simulink model "gm_base_band_shaping_model_fil"  (R2020b)
settings: Solver=FixedStepDiscrete  StartTime=0.0  StopTime=400  RelTol=1e-3
libraries: simulink x2, dspmlti4 x2, whdlio x1, commdigbbndpm3 x1, commrandsrc3 x1, fillib x1
settings Model: Creator=wardo  LastModifiedBy=wardo
settings DataIOCC: LimitDataPoints=on  SaveOutput=off  SaveTime=off
settings OptimizationCC: BlockReduction=off  ConditionallyExecuteInputs=off  DefaultParameterBehavior=Inlined  LifeSpan=inf
settings DebuggingCC: AlgebraicLoopMsg=error  InheritedTsInSrcMsg=none  SingleTaskRateTransMsg=error  AllowSymbolicDim=off  StrictBusMsg=ErrorOnBusTreatedAsVector  SFUnexpectedBacktrackingDiag=warning  SFNoUnconditionalDefaultTransitionDiag=warning  SFExecutionAtInitializationDiag=none  ArithmeticOperatorsInVariantConditions=warning
settings HardwareCC: ProdBitPerPointer=32  ProdBitPerSizeT=32  ProdBitPerPtrDiffT=32  ProdLargestAtomicFloat=None  ProdIntDivRoundTo=Undefined  ProdEndianess=Unspecified  ProdWordSize=32  ProdHWDeviceType=ASIC/FPGA->ASIC/FPGA  ProdEqTarget=off
settings SFSimCC: SimUseLocalCustomCode=off  CustomCodeUndefinedFunction=UseInterfaceOnly
settings RTWCC: RTWUseLocalCustomCode=off
settings CodeAppCC: StateflowObjectComments=on
settings GRTTargetCC: TargetLangStandard=C89/C90 (ANSI)
settings ConfigComp: CovScope=ReferencedModels  CovMetricSettings=dw  CovSaveCumulativeToWorkspaceVar=on  CovSaveSingleToWorkspaceVar=on  CovExternalEMLEnable=off  CovSFcnEnable=off

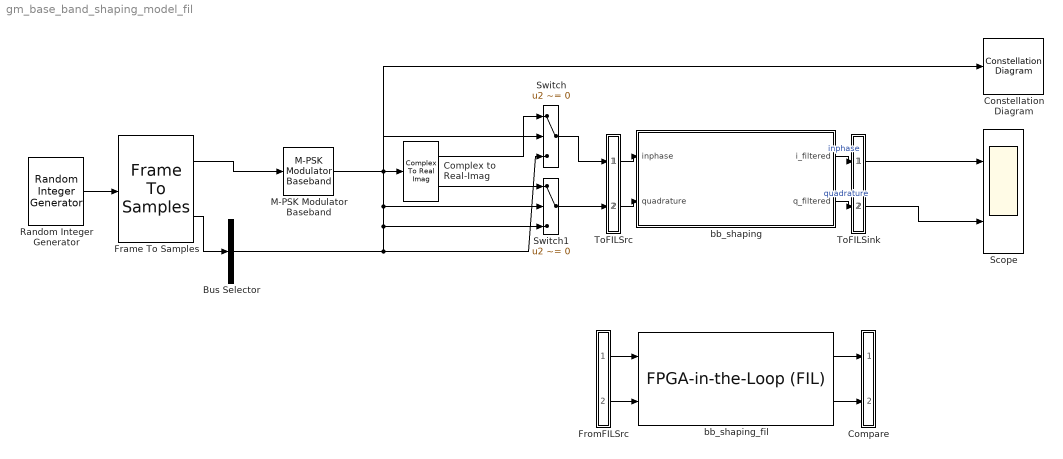
== system gm_base_band_shaping_model_fil ==
  Bus Selector : BusSelector  OutputSignals=valid
  Compare : Subsystem
      mask Display: disp('')
  Complex to Real-Imag : ComplexToRealImag
  Constellation Diagram : ConstellationDiagram
  Frame To Samples : whdlio/Frame To Samples  InterSampleIdleCycles=1  InterFrameIdleCycles=100  OutputSize=1  InterleaveSamples=off
      settings: SourceProductBaseCode=LH
  FromFILSrc : Subsystem
      mask Display: disp('')
  M-PSK Modulator Baseband : commdigbbndpm3/M-PSK Modulator Baseband  M=8  InType=Integer  Enc=Gray  Mapping=[0:7]  Ph=0  outDtype=Fixed-point  outWordLen=18  outUDDataType=sfix(16)  outFracLenMode=User-defined  outFracLen=14  outDataTypeStr=fixdt(1,18,14)  outLastDataTypeStr=fixdt(1,18,14)
      settings: SourceProductName=Communications Toolbox
  Random Integer Generator : commrandsrc3/Random Integer Generator  SetSize=8  SeedSource=Auto  Seed=0  SampleTime=10  SamplesPerFrame=10  OutputDataType=double  SimulateUsing=Interpreted execution
  Scope : Scope  NumInputPorts=2
  Switch : Switch  Criteria=u2 ~= 0  OutDataTypeStr=Inherit: Inherit via back propagation
  Switch1 : Switch  Criteria=u2 ~= 0  OutDataTypeStr=Inherit: Inherit via back propagation
  ToFILSink : Subsystem
      mask Display: disp('')
  ToFILSrc : Subsystem
      mask Display: disp('')
  bb_shaping : Subsystem
  bb_shaping_fil : fillib/FPGA-in-the-Loop (FIL)  ForceInterfaceUpdate=0.43904
      settings: SourceProductBaseCode=ES,HD
  wires:
  Frame To Samples/1 -> M-PSK Modulator Baseband/1
  M-PSK Modulator Baseband/1 -> Complex to Real-Imag/1, Constellation Diagram/1
  Random Integer Generator/1 -> Frame To Samples/1
  Frame To Samples/2 -> Bus Selector/1
  Bus Selector/1 -> Switch/2, Switch1/2, Switch1/3, Switch/3
  Complex to Real-Imag/1 -> Switch/1
  Complex to Real-Imag/2 -> Switch1/1
  ToFILSrc/1(out1) -> bb_shaping/1(inphase)
  ToFILSrc/2(out2) -> bb_shaping/2(quadrature)
  bb_shaping/1(i_filtered) -> ToFILSink/1(in1)  "inphase"
  bb_shaping/2(q_filtered) -> ToFILSink/2(in2)  "quadrature"
  Switch/1 -> ToFILSrc/1(in1)
  Switch1/1 -> ToFILSrc/2(in2)
  ToFILSink/1(out1) -> Scope/1
  ToFILSink/2(out2) -> Scope/2
  FromFILSrc/1(out1) -> bb_shaping_fil/1
  FromFILSrc/2(out2) -> bb_shaping_fil/2
  bb_shaping_fil/1 -> Compare/1(in1)
  bb_shaping_fil/2 -> Compare/2(in2)

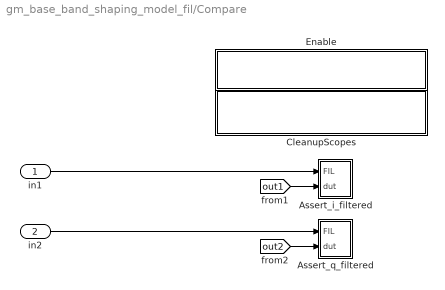
== system gm_base_band_shaping_model_fil/Compare ==
  in1 : Inport
  in2 : Inport  Port=2
  Assert_i_filtered : Subsystem
  Assert_q_filtered : Subsystem
  CleanupScopes : Subsystem
      settings: OpenFcn=|
      | blkName = gcb; %self block
      | idx = regexp(blkName, '/CleanupScopes$', 'once');
      | blkParent = blkName(1:idx-1);
      | blks=find_system(blkParent, 'LookUnderMasks', 'all','blocktype', 'Scope');
      | for itr = 1:length(blks)
      | 	 hScopeCfg = get_param(blks{itr},'ScopeConfiguration');
      | 	 hScopeCfg.Visible = ~ hScopeCfg.Visible;
      | end
      | drawnow;
      mask Display: fprintf(message('hdlcoder:cosim:vnl_dblclick').getString());
  Enable : Subsystem
      settings: OpenFcn=|
      | blkName = gcb;
      | idx = regexp(blkName, '/Enable$', 'once');
      | blkParent = blkName(1:idx-1);
      | blks=find_system(blkParent, 'LookUnderMasks', 'all','blocktype', 'Assertion');
      | e = get_param(blks{1}, 'Enabled');
      | if strcmp(e, 'on'), f= 'off';, else, f = 'on';, end
      | for ii=1:length(blks), set_param(blks{ii}, 'Enabled', f);, end
      | set_param(gcb, 'MaskDisplay',['fprintf(message(''hdlcoder:cosim:vnl_dblclick_assertions'',','''',upper(e),'''',').getString())']);
      mask Display: fprintf(message('hdlcoder:cosim:vnl_dblclick_assertions','OFF').getString());
  wires:
  in1/1 -> Assert_i_filtered/1(FIL)
  [out1] -> Assert_i_filtered/2(dut)
  in2/1 -> Assert_q_filtered/1(FIL)
  [out2] -> Assert_q_filtered/2(dut)

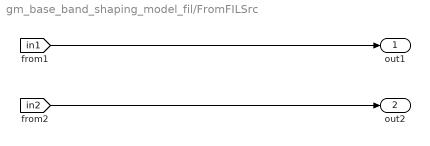
== system gm_base_band_shaping_model_fil/FromFILSrc ==
  out1 : Outport
  out2 : Outport  Port=2
  wires:
  [in1] -> out1/1
  [in2] -> out2/1

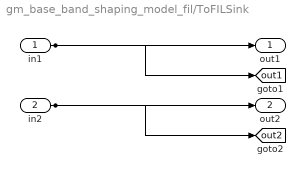
== system gm_base_band_shaping_model_fil/ToFILSink ==
  in1 : Inport
  in2 : Inport  Port=2
  out1 : Outport
  out2 : Outport  Port=2
  tag scope: out1=global, out2=global
  wires:
  in1/1 -> out1/1, [out1]
  in2/1 -> out2/1, [out2]

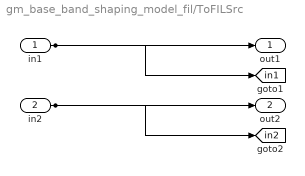
== system gm_base_band_shaping_model_fil/ToFILSrc ==
  in1 : Inport
  in2 : Inport  Port=2
  out1 : Outport
  out2 : Outport  Port=2
  tag scope: in1=global, in2=global
  wires:
  in1/1 -> out1/1, [in1]
  in2/1 -> out2/1, [in2]

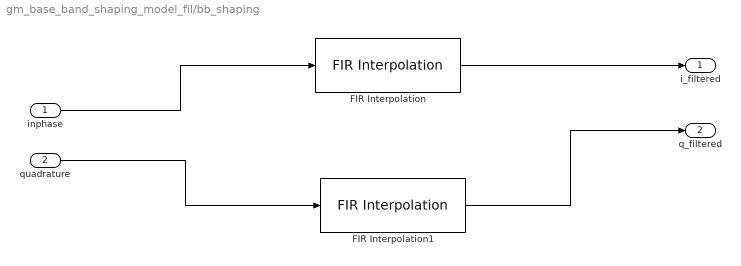
== system gm_base_band_shaping_model_fil/bb_shaping ==
  inphase : Inport  OutDataTypeStr=fixdt(1, 18, 14)  PortDimensions=1  SampleTime=0.833333333333333
  quadrature : Inport  Port=2  OutDataTypeStr=fixdt(1, 18, 14)  PortDimensions=1  SampleTime=0.833333333333333
  FIR Interpolation : dspmlti4/FIR Interpolation  FilterSource=Dialog parameters  PrivateCoeffs=0  h=[-0.00599670410156250,-0.00514221191406250,-0.00289916992187500,0.000442504882812500,0.00431823730468750,0.00794982910156250,0.0104980468750000,0.0112304687500000,0.00967407226562500,0.00578308105468750,0,-0.00680541992187500,-0.0134124755859375,-0.0184326171875000,-0.0205841064453125,-0.0189819335937500,-0.0133361816406250,-0.00410461425781250,0.00752258300781250,0.0196380615234375,0.0300140380859375,0.0363464355468750,0.0367584228515625,0.0301208496093750,0.0164794921875000,-0.00291442871093750,-0.0254821777343750,-0.0476837158203125,-0.0653228759765625,-0.0742187500000000,-0.0707244873046875,-0.0524291992187500,-0.0185852050781250,0.0296783447265625,0.0892028808593750,0.155227661132813,0.221755981445313,0.282333374023438,0.330810546875000,0.362121582031250,0.372940063476563,0.362121582031250,0.330810546875000,0.282333374023438,0.221755981445313,0.155227661132813,0.0892028808593750,0.0296783447265625,-0.0185852050781250,-0.0524291992187500,-0.0707244873046875,-0.0742187500000000,-0.0653228759765625,-0.0476837158203125,-0.0254821777343750,-0.00291442871093750,0.0164794921875000,0.0301208496093750,0.0367584228515625,0.0363464355468750,0.0300140380859375,0.0196380615234375,0.00752258300781250,-0.00410461425781250,-0.0133361816406250,-0.0189819335937500,-0.0205841064453125,-0.0184326171875000,-0.0134124755859375,-0.00680541992187500,0,0.00578308105468750,0.00967407226562500,0.0112304687500000,0.0104980468750000,0.00794982910156250,0.00431823730468750,0.000442504882812500,-0.00289916992187500,-0.00514221191406250,-0.00599670410156250]  L=8  FilterObject=FINTERP  framing=Allow multirate processing  outputBufInitCond=0  roundingMode=Floor  overflowMode=off  firstCoeffMode=Specify word length  firstCoeffWordLength=16  firstCoeffFracLength=15  firstCoeffDataTypeStr=fixdt(1,16)  firstCoeffMin=[]  firstCoeffMax=[]  firstCoeffLastDataTypeStr=fixdt(1,16)  outputDataTypeStr=Inherit: Same as accumulator  outputMin=[]  outputMax=[]  outputLastDataTypeStr=Inherit: Same as accumulator
      settings: SourceProductName=DSP System Toolbox
  FIR Interpolation1 : dspmlti4/FIR Interpolation  FilterSource=Dialog parameters  PrivateCoeffs=0  h=[-0.00599670410156250,-0.00514221191406250,-0.00289916992187500,0.000442504882812500,0.00431823730468750,0.00794982910156250,0.0104980468750000,0.0112304687500000,0.00967407226562500,0.00578308105468750,0,-0.00680541992187500,-0.0134124755859375,-0.0184326171875000,-0.0205841064453125,-0.0189819335937500,-0.0133361816406250,-0.00410461425781250,0.00752258300781250,0.0196380615234375,0.0300140380859375,0.0363464355468750,0.0367584228515625,0.0301208496093750,0.0164794921875000,-0.00291442871093750,-0.0254821777343750,-0.0476837158203125,-0.0653228759765625,-0.0742187500000000,-0.0707244873046875,-0.0524291992187500,-0.0185852050781250,0.0296783447265625,0.0892028808593750,0.155227661132813,0.221755981445313,0.282333374023438,0.330810546875000,0.362121582031250,0.372940063476563,0.362121582031250,0.330810546875000,0.282333374023438,0.221755981445313,0.155227661132813,0.0892028808593750,0.0296783447265625,-0.0185852050781250,-0.0524291992187500,-0.0707244873046875,-0.0742187500000000,-0.0653228759765625,-0.0476837158203125,-0.0254821777343750,-0.00291442871093750,0.0164794921875000,0.0301208496093750,0.0367584228515625,0.0363464355468750,0.0300140380859375,0.0196380615234375,0.00752258300781250,-0.00410461425781250,-0.0133361816406250,-0.0189819335937500,-0.0205841064453125,-0.0184326171875000,-0.0134124755859375,-0.00680541992187500,0,0.00578308105468750,0.00967407226562500,0.0112304687500000,0.0104980468750000,0.00794982910156250,0.00431823730468750,0.000442504882812500,-0.00289916992187500,-0.00514221191406250,-0.00599670410156250]  L=8  FilterObject=FINTERP  framing=Allow multirate processing  outputBufInitCond=0  roundingMode=Floor  overflowMode=off  firstCoeffMode=Specify word length  firstCoeffWordLength=16  firstCoeffFracLength=15  firstCoeffDataTypeStr=fixdt(1,16)  firstCoeffMin=[]  firstCoeffMax=[]  firstCoeffLastDataTypeStr=fixdt(1,16)  outputDataTypeStr=Inherit: Same as accumulator  outputMin=[]  outputMax=[]  outputLastDataTypeStr=Inherit: Same as accumulator
      settings: SourceProductName=DSP System Toolbox
  i_filtered : Outport  VectorParamsAs1DForOutWhenUnconnected=off
  q_filtered : Outport  Port=2  VectorParamsAs1DForOutWhenUnconnected=off
  wires:
  FIR Interpolation1/1 -> q_filtered/1
  FIR Interpolation/1 -> i_filtered/1
  quadrature/1 -> FIR Interpolation1/1
  inphase/1 -> FIR Interpolation/1

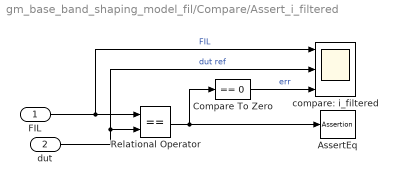
== system gm_base_band_shaping_model_fil/Compare/Assert_i_filtered ==
  FIL : Inport
  dut : Inport  Port=2
  AssertEq : Assertion  StopWhenAssertionFail=off
  Compare To Zero : simulink/Logic and Bit Operations/Compare To Zero  relop===  OutDataTypeStr=boolean
  Relational Operator : RelationalOperator  Operator===  OutDataTypeStr=boolean  RndMeth=Nearest
  compare: i_filtered : Scope  NumInputPorts=3
  wires:
  Compare To Zero/1 -> compare: i_filtered/3  "err"
  Relational Operator/1 -> Compare To Zero/1, AssertEq/1
  FIL/1 -> compare: i_filtered/1, Relational Operator/1  "FIL"
  dut/1 -> compare: i_filtered/2, Relational Operator/2  "dut ref"

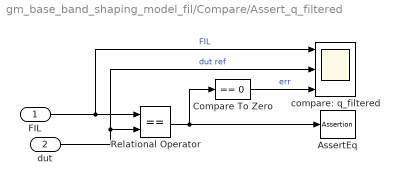
== system gm_base_band_shaping_model_fil/Compare/Assert_q_filtered ==
  FIL : Inport
  dut : Inport  Port=2
  AssertEq : Assertion  StopWhenAssertionFail=off
  Compare To Zero : simulink/Logic and Bit Operations/Compare To Zero  relop===  OutDataTypeStr=boolean
  Relational Operator : RelationalOperator  Operator===  OutDataTypeStr=boolean  RndMeth=Nearest
  compare: q_filtered : Scope  NumInputPorts=3
  wires:
  Compare To Zero/1 -> compare: q_filtered/3  "err"
  Relational Operator/1 -> Compare To Zero/1, AssertEq/1
  FIL/1 -> compare: q_filtered/1, Relational Operator/1  "FIL"
  dut/1 -> compare: q_filtered/2, Relational Operator/2  "dut ref"

== system gm_base_band_shaping_model_fil/Compare/CleanupScopes ==

== system gm_base_band_shaping_model_fil/Compare/Enable ==
